simulink model "LWR"  (R2018b)
settings: Solver=FixedStepAuto  StartTime=0.0  StopTime=10  FixedStep=0.01  RelTol=1e-3
model workspace: external: MATLAB File F:\Research\AAA\LWR_DataFile.m (data not in the file)
values from neighbouring files (symbols this model uses):
  m = max([i j])    [Dynamic_model_eq.m]
  robot = robotics.RigidBodyTree("MaxNumBodies",8,"DataFormat","row")    [RigidBodyTree.m]
undefined symbols (not defined in the file or in its folder): smiData, X, Y, Z
libraries: sm_lib x86, fl_lib x42, nesl_utility x36, elec_lib x21, dspmtrx3 x7, robotmaniplib x2
(part 1 of 3)
settings Model: Creator=Cristian  LastModifiedBy=Cristian

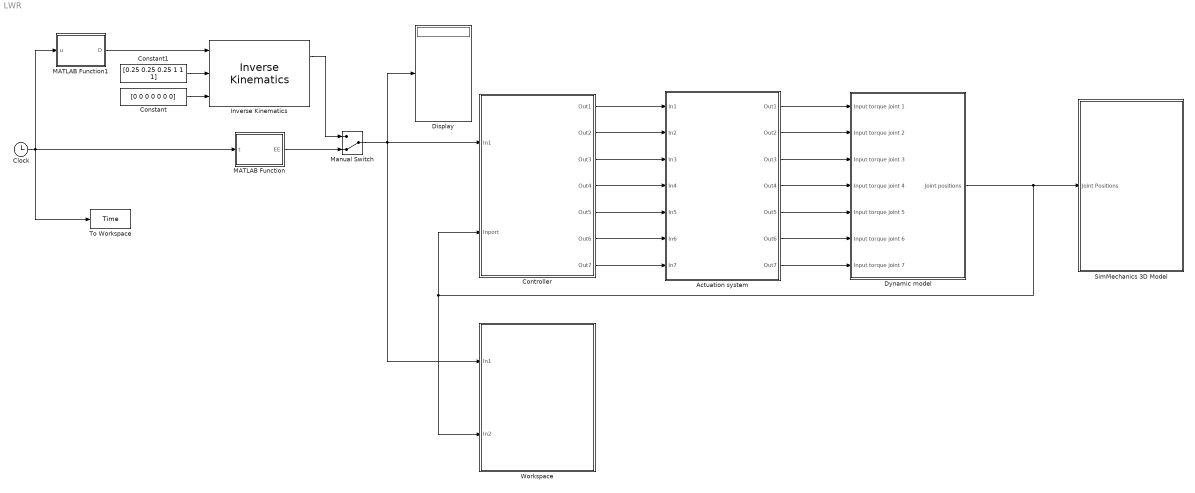
== system LWR ==
  Actuation system : Subsystem
  Clock : Clock
  Constant : Constant  Value=[0 0 0 0 0 0 0]
  Constant1 : Constant  Value=[0.25 0.25 0.25 1 1 1]
  Controller : Subsystem
  Display : Display
  "Dynamic model " : Subsystem
  Inverse Kinematics : robotmaniplib/Inverse Kinematics  RigidBodyTree=robot  EndEffector=body7  ShowInfo=on  SolverName=BFGS Gradient Projection  EnforceJointLimits=on  MaxIterations=1500  MaxTime=10  GradientTolerance=1e-7  SolutionTolerance=1e-6  StepTolerance=1e-14  ErrorChangeTolerance=1e-12  UseErrorDamping=on  DampingBias=0.0025
      settings: SourceProductName=Robotics System Toolbox
  MATLAB Function : MATLAB Function  TreatAsAtomicUnit=on
  MATLAB Function1 : MATLAB Function  TreatAsAtomicUnit=on
  Manual Switch : ManualSwitch  CurrentSetting=0
  SimMechanics 3D Model : Subsystem
      mask Display: image('photo1.jpg');
  To Workspace : ToWorkspace  VariableName=Time  SampleTime=-1
  Workspace : Subsystem
  wires:
  "Dynamic model "/1(Joint positions) -> Controller/2(Inport), Workspace/2(In2), SimMechanics 3D Model/1(Joint Positions)
  Controller/1(Out1) -> Actuation system/1(In1)
  Controller/2(Out2) -> Actuation system/2(In2)
  Controller/3(Out3) -> Actuation system/3(In3)
  Controller/4(Out4) -> Actuation system/4(In4)
  Controller/5(Out5) -> Actuation system/5(In5)
  Controller/6(Out6) -> Actuation system/6(In6)
  Controller/7(Out7) -> Actuation system/7(In7)
  Actuation system/1(Out1) -> "Dynamic model "/1(Input torque joint 1)
  Actuation system/2(Out2) -> "Dynamic model "/2(Input torque joint 2)
  Actuation system/3(Out3) -> "Dynamic model "/3(Input torque joint 3)
  Actuation system/4(Out4) -> "Dynamic model "/4(Input torque joint 4)
  Actuation system/5(Out5) -> "Dynamic model "/5(Input torque joint 5)
  Actuation system/6(Out6) -> "Dynamic model "/6(Input torque joint 6)
  Actuation system/7(Out7) -> "Dynamic model "/7(Input torque joint 7)
  Clock/1 -> To Workspace/1, MATLAB Function/1(t), MATLAB Function1/1(u)
  Manual Switch/1 -> Display/1, Workspace/1(In1), Controller/1(In1)
  MATLAB Function/1(EE) -> Manual Switch/2
  Constant/1 -> Inverse Kinematics/3
  Constant1/1 -> Inverse Kinematics/2
  MATLAB Function1/1(O) -> Inverse Kinematics/1
  Inverse Kinematics/1 -> Manual Switch/1

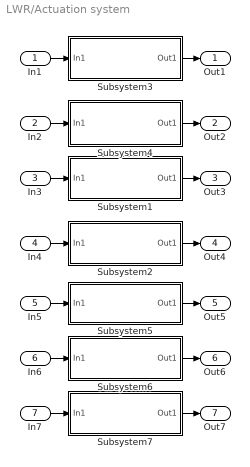
== system LWR/Actuation system ==
  In1 : Inport
  In2 : Inport  Port=2
  In3 : Inport  Port=3
  In4 : Inport  Port=4
  In5 : Inport  Port=5
  In6 : Inport  Port=6
  In7 : Inport  Port=7
  Subsystem1 : Subsystem
  Subsystem2 : Subsystem
  Subsystem3 : Subsystem
  Subsystem4 : Subsystem
  Subsystem5 : Subsystem
  Subsystem6 : Subsystem
  Subsystem7 : Subsystem
  Out1 : Outport
  Out2 : Outport  Port=2
  Out3 : Outport  Port=3
  Out4 : Outport  Port=4
  Out5 : Outport  Port=5
  Out6 : Outport  Port=6
  Out7 : Outport  Port=7
  wires:
  In2/1 -> Subsystem4/1(In1)
  In3/1 -> Subsystem1/1(In1)
  Subsystem7/1(Out1) -> Out7/1
  In1/1 -> Subsystem3/1(In1)
  In5/1 -> Subsystem5/1(In1)
  Subsystem1/1(Out1) -> Out3/1
  Subsystem5/1(Out1) -> Out5/1
  Subsystem4/1(Out1) -> Out2/1
  Subsystem3/1(Out1) -> Out1/1
  In6/1 -> Subsystem6/1(In1)
  Subsystem2/1(Out1) -> Out4/1
  Subsystem6/1(Out1) -> Out6/1
  In4/1 -> Subsystem2/1(In1)
  In7/1 -> Subsystem7/1(In1)

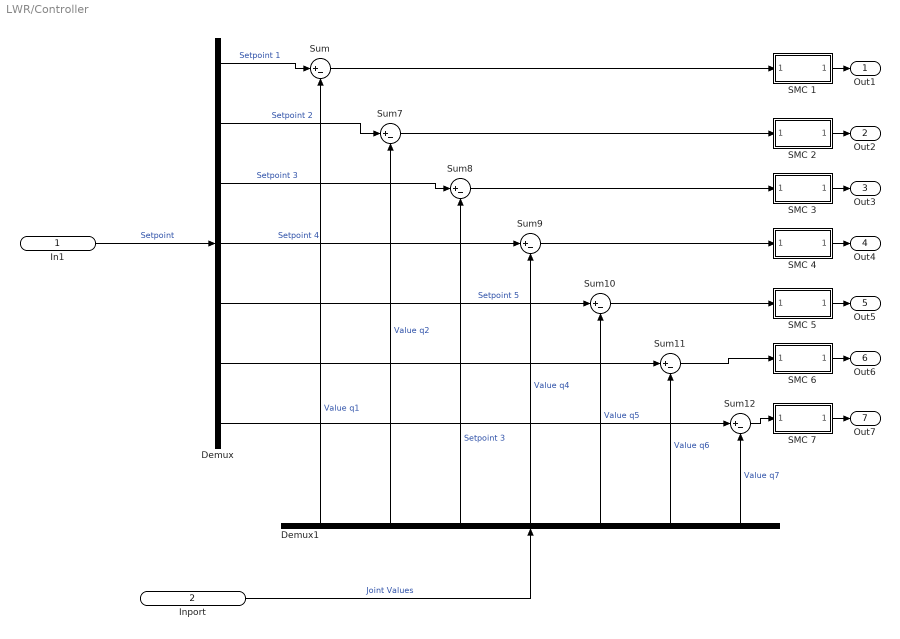
== system LWR/Controller ==
  In1 : Inport
  Inport : Inport  Port=2
  Demux : Demux  Outputs=7
  Demux1 : Demux  Outputs=7
  SMC 1 : Subsystem
  SMC 2 : Subsystem
  SMC 3 : Subsystem
  SMC 4 : Subsystem
  SMC 5 : Subsystem
  SMC 6 : Subsystem
  SMC 7 : Subsystem
  Sum{,7..12} (7 alike) : Sum  Inputs=|+-
  Out1 : Outport
  Out2 : Outport  Port=2
  Out3 : Outport  Port=3
  Out4 : Outport  Port=4
  Out5 : Outport  Port=5
  Out6 : Outport  Port=6
  Out7 : Outport  Port=7
  wires:
  Sum/1 -> SMC 1/1(error)
  Sum9/1 -> SMC 4/1(error)
  Sum8/1 -> SMC 3/1(error)
  Demux1/6 -> Sum11/2  "Value q6"
  Demux1/1 -> Sum/2  "Value q1"
  Demux/1 -> Sum/1  "Setpoint 1"
  Demux1/5 -> Sum10/2  "Value q5"
  Sum7/1 -> SMC 2/1(error)
  SMC 5/1(Out1) -> Out5/1
  Sum10/1 -> SMC 5/1(error)
  Sum11/1 -> SMC 6/1(error)
  Sum12/1 -> SMC 7/1(error)
  Demux/2 -> Sum7/1  "Setpoint 2"
  Demux/3 -> Sum8/1  "Setpoint 3"
  Demux1/4 -> Sum9/2  "Value q4"
  SMC 6/1(Out1) -> Out6/1
  SMC 4/1(Out1) -> Out4/1
  Demux/5 -> Sum10/1  "Setpoint 5"
  Demux1/2 -> Sum7/2  "Value q2"
  Demux1/3 -> Sum8/2  "Setpoint 3"
  Demux/4 -> Sum9/1  "Setpoint 4"
  SMC 2/1(Out1) -> Out2/1
  SMC 7/1(Out1) -> Out7/1
  Demux1/7 -> Sum12/2  "Value q7"
  SMC 3/1(Out1) -> Out3/1
  SMC 1/1(Out1) -> Out1/1
  Inport/1 -> Demux1/1  "Joint Values"
  In1/1 -> Demux/1  "Setpoint"
  Demux/6 -> Sum11/1
  Demux/7 -> Sum12/1

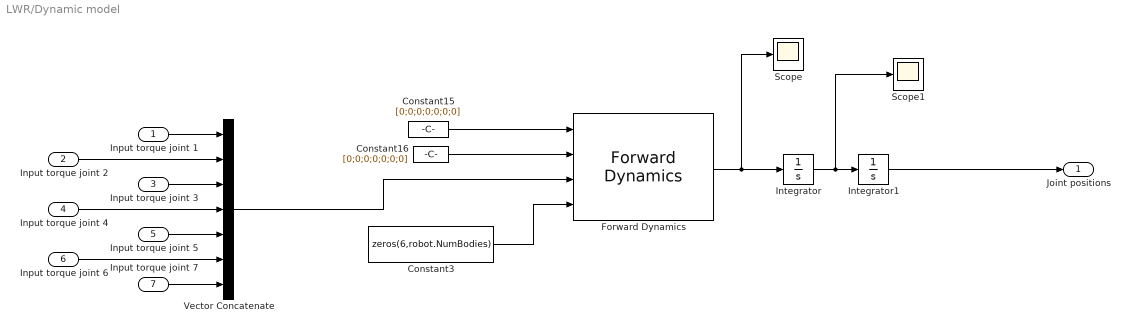
== system LWR/Dynamic model  ==
  Input torque joint 1 : Inport
  Input torque joint 2 : Inport  Port=2
  Input torque joint 3 : Inport  Port=3
  Input torque joint 4 : Inport  Port=4
  Input torque joint 5 : Inport  Port=5
  Input torque joint 6 : Inport  Port=6
  Input torque joint 7 : Inport  Port=7
  Constant15 : Constant  Value=[0;0;0;0;0;0;0]
  Constant16 : Constant  Value=[0;0;0;0;0;0;0]
  Constant3 : Constant  Value=zeros(6,robot.NumBodies)
  Forward Dynamics : robotmaniplib/Forward Dynamics  RigidBodyTree=robot
      settings: SourceProductName=Robotics System Toolbox
  Integrator : Integrator
  Integrator1 : Integrator
  Scope : Scope
  Scope1 : Scope
  Vector Concatenate : Concatenate  NumInputs=7
  Joint positions : Outport
  wires:
  Constant16/1 -> Forward Dynamics/2
  Forward Dynamics/1 -> Scope/1, Integrator/1
  Constant15/1 -> Forward Dynamics/1
  Integrator/1 -> Scope1/1, Integrator1/1
  Integrator1/1 -> Joint positions/1
  Vector Concatenate/1 -> Forward Dynamics/3
  Constant3/1 -> Forward Dynamics/4
  Input torque joint 1/1 -> Vector Concatenate/1
  Input torque joint 2/1 -> Vector Concatenate/2
  Input torque joint 3/1 -> Vector Concatenate/3
  Input torque joint 4/1 -> Vector Concatenate/4
  Input torque joint 5/1 -> Vector Concatenate/5
  Input torque joint 6/1 -> Vector Concatenate/6
  Input torque joint 7/1 -> Vector Concatenate/7

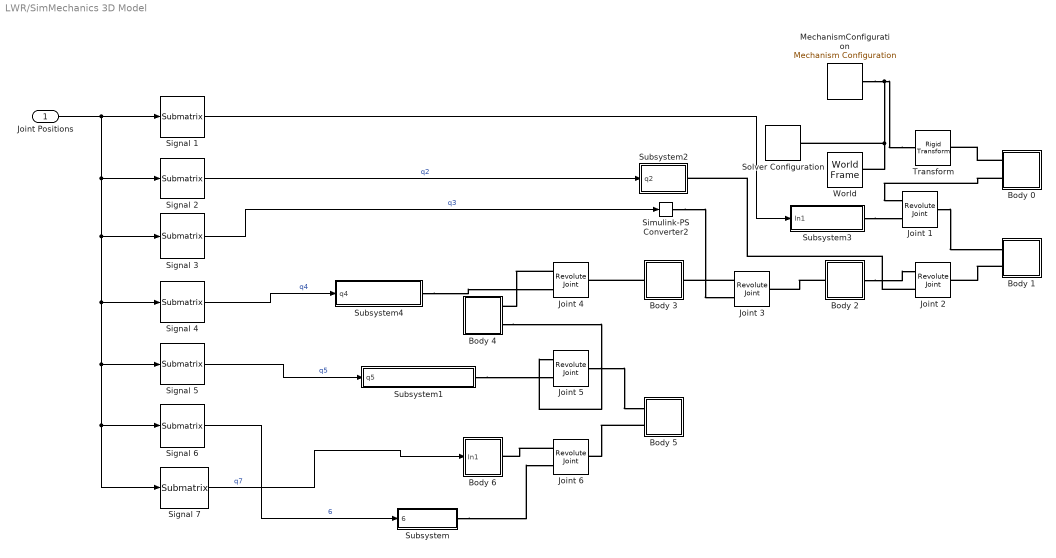
== system LWR/SimMechanics 3D Model ==
  Joint Positions : Inport
  Body 0 : Subsystem
  Body 1 : Subsystem
  Body 2 : Subsystem
  Body 3 : Subsystem
  Body 4 : Subsystem
  Body 5 : Subsystem
  Body 6 : Subsystem
  Joint 1 : sm_lib/Joints/Revolute Joint  SenseConstraintForce=off  SenseConstraintForceX=off  SenseConstraintForceY=off  SenseConstraintForceZ=off  SenseConstraintTorque=off  SenseConstraintTorqueX=off  SenseConstraintTorqueY=off  SenseConstraintTorqueZ=off  SenseTotalForce=off  SenseTotalForceX=off  SenseTotalForceY=off  SenseTotalForceZ=off  SenseTotalTorque=off  SenseTotalTorqueX=off  SenseTotalTorqueY=off  SenseTotalTorqueZ=off  CompositeWrenchDir=FollowerOnBase  CompositeWrenchFrame=BaseFrame  EquilibriumPosition=0  EquilibriumPositionUnits=rad  SpringStiffness=0  SpringStiffnessUnits=N*m/rad  DampingCoefficient=0  DampingCoefficientUnits=N*m/(rad/s)  TorqueActuationMode=ComputedTorque  MotionActuationMode=InputMotion  SensePosition=off  SenseVelocity=off  SenseAcceleration=off  SenseTorqueForce=off  PositionTargetSpecify=on  PositionTargetPriority=High  PositionTargetValue=2.094395  PositionTargetValueUnits=rad  VelocityTargetSpecify=on  VelocityTargetPriority=High  VelocityTargetValue=0  VelocityTargetValueUnits=deg/s
  Joint 2 : sm_lib/Joints/Revolute Joint  SenseConstraintForce=off  SenseConstraintForceX=off  SenseConstraintForceY=off  SenseConstraintForceZ=off  SenseConstraintTorque=off  SenseConstraintTorqueX=off  SenseConstraintTorqueY=off  SenseConstraintTorqueZ=off  SenseTotalForce=off  SenseTotalForceX=off  SenseTotalForceY=off  SenseTotalForceZ=off  SenseTotalTorque=off  SenseTotalTorqueX=off  SenseTotalTorqueY=off  SenseTotalTorqueZ=off  CompositeWrenchDir=FollowerOnBase  CompositeWrenchFrame=BaseFrame  EquilibriumPosition=0  EquilibriumPositionUnits=rad  SpringStiffness=0  SpringStiffnessUnits=N*m/rad  DampingCoefficient=0  DampingCoefficientUnits=N*m/(rad/s)  TorqueActuationMode=ComputedTorque  MotionActuationMode=InputMotion  SensePosition=off  SenseVelocity=off  SenseAcceleration=off  SenseTorqueForce=off  PositionTargetSpecify=on  PositionTargetPriority=High  PositionTargetValue=5.9341  PositionTargetValueUnits=rad  VelocityTargetSpecify=on  VelocityTargetPriority=High  VelocityTargetValue=0  VelocityTargetValueUnits=deg/s
  Joint 3 : sm_lib/Joints/Revolute Joint  SenseConstraintForce=off  SenseConstraintForceX=off  SenseConstraintForceY=off  SenseConstraintForceZ=off  SenseConstraintTorque=off  SenseConstraintTorqueX=off  SenseConstraintTorqueY=off  SenseConstraintTorqueZ=off  SenseTotalForce=off  SenseTotalForceX=off  SenseTotalForceY=off  SenseTotalForceZ=off  SenseTotalTorque=off  SenseTotalTorqueX=off  SenseTotalTorqueY=off  SenseTotalTorqueZ=off  CompositeWrenchDir=FollowerOnBase  CompositeWrenchFrame=BaseFrame  EquilibriumPosition=0  EquilibriumPositionUnits=rad  SpringStiffness=0  SpringStiffnessUnits=N*m/rad  DampingCoefficient=0  DampingCoefficientUnits=N*m/(rad/s)  TorqueActuationMode=ComputedTorque  MotionActuationMode=InputMotion  SensePosition=off  SenseVelocity=off  SenseAcceleration=off  SenseTorqueForce=off  PositionTargetSpecify=on  PositionTargetPriority=High  PositionTargetValue=0  PositionTargetValueUnits=deg  VelocityTargetSpecify=off  VelocityTargetPriority=High  VelocityTargetValue=0  VelocityTargetValueUnits=deg/s
  Joint 4 : sm_lib/Joints/Revolute Joint  SenseConstraintForce=off  SenseConstraintForceX=off  SenseConstraintForceY=off  SenseConstraintForceZ=off  SenseConstraintTorque=off  SenseConstraintTorqueX=off  SenseConstraintTorqueY=off  SenseConstraintTorqueZ=off  SenseTotalForce=off  SenseTotalForceX=off  SenseTotalForceY=off  SenseTotalForceZ=off  SenseTotalTorque=off  SenseTotalTorqueX=off  SenseTotalTorqueY=off  SenseTotalTorqueZ=off  CompositeWrenchDir=FollowerOnBase  CompositeWrenchFrame=BaseFrame  EquilibriumPosition=0  EquilibriumPositionUnits=rad  SpringStiffness=0  SpringStiffnessUnits=N*m/rad  DampingCoefficient=0  DampingCoefficientUnits=N*m/(rad/s)  TorqueActuationMode=ComputedTorque  MotionActuationMode=InputMotion  SensePosition=off  SenseVelocity=off  SenseAcceleration=off  SenseTorqueForce=off  PositionTargetSpecify=on  PositionTargetPriority=High  PositionTargetValue=4.8869  PositionTargetValueUnits=rad  VelocityTargetSpecify=off  VelocityTargetPriority=High  VelocityTargetValue=0  VelocityTargetValueUnits=deg/s
  Joint 5 : sm_lib/Joints/Revolute Joint  SenseConstraintForce=off  SenseConstraintForceX=off  SenseConstraintForceY=off  SenseConstraintForceZ=off  SenseConstraintTorque=off  SenseConstraintTorqueX=off  SenseConstraintTorqueY=off  SenseConstraintTorqueZ=off  SenseTotalForce=off  SenseTotalForceX=off  SenseTotalForceY=off  SenseTotalForceZ=off  SenseTotalTorque=off  SenseTotalTorqueX=off  SenseTotalTorqueY=off  SenseTotalTorqueZ=off  CompositeWrenchDir=FollowerOnBase  CompositeWrenchFrame=BaseFrame  EquilibriumPosition=0  EquilibriumPositionUnits=rad  SpringStiffness=0  SpringStiffnessUnits=N*m/rad  DampingCoefficient=0  DampingCoefficientUnits=N*m/(rad/s)  TorqueActuationMode=ComputedTorque  MotionActuationMode=InputMotion  SensePosition=off  SenseVelocity=off  SenseAcceleration=off  SenseTorqueForce=off  PositionTargetSpecify=on  PositionTargetPriority=High  PositionTargetValue=0.349  PositionTargetValueUnits=rad  VelocityTargetSpecify=off  VelocityTargetPriority=High  VelocityTargetValue=0  VelocityTargetValueUnits=deg/s
  Joint 6 : sm_lib/Joints/Revolute Joint  SenseConstraintForce=off  SenseConstraintForceX=off  SenseConstraintForceY=off  SenseConstraintForceZ=off  SenseConstraintTorque=off  SenseConstraintTorqueX=off  SenseConstraintTorqueY=off  SenseConstraintTorqueZ=off  SenseTotalForce=off  SenseTotalForceX=off  SenseTotalForceY=off  SenseTotalForceZ=off  SenseTotalTorque=off  SenseTotalTorqueX=off  SenseTotalTorqueY=off  SenseTotalTorqueZ=off  CompositeWrenchDir=FollowerOnBase  CompositeWrenchFrame=BaseFrame  EquilibriumPosition=0  EquilibriumPositionUnits=rad  SpringStiffness=0  SpringStiffnessUnits=N*m/rad  DampingCoefficient=0  DampingCoefficientUnits=N*m/(rad/s)  TorqueActuationMode=ComputedTorque  MotionActuationMode=InputMotion  SensePosition=off  SenseVelocity=off  SenseAcceleration=off  SenseTorqueForce=off  PositionTargetSpecify=on  PositionTargetPriority=Low  PositionTargetValue=0.2617  PositionTargetValueUnits=rad  VelocityTargetSpecify=off  VelocityTargetPriority=High  VelocityTargetValue=0  VelocityTargetValueUnits=deg/s
  MechanismConfiguration : sm_lib/Utilities/Mechanism Configuration  UniformGravity=Constant  GravityVector=[0 -9.80665 0]  GravityUnits=m/s^2  LinearizationDelta=0.001
  Signal 1 : dspmtrx3/Submatrix  RowSpan=One row  RowStartMode=First  RowStartIndex=1  RowEndMode=Last  RowEndIndex=1  ColSpan=One column  ColStartMode=First  ColStartIndex=1  ColEndMode=Last  ColEndIndex=1
  Signal 2 : dspmtrx3/Submatrix  RowSpan=One row  RowStartMode=Index  RowStartIndex=2  RowEndMode=Last  RowEndIndex=1  ColSpan=One column  ColStartMode=First  ColStartIndex=1  ColEndMode=Last  ColEndIndex=1
  Signal 3 : dspmtrx3/Submatrix  RowSpan=One row  RowStartMode=Index  RowStartIndex=3  RowEndMode=Last  RowEndIndex=1  ColSpan=One column  ColStartMode=First  ColStartIndex=1  ColEndMode=Last  ColEndIndex=1
  Signal 4 : dspmtrx3/Submatrix  RowSpan=One row  RowStartMode=Index  RowStartIndex=4  RowEndMode=Last  RowEndIndex=1  ColSpan=One column  ColStartMode=First  ColStartIndex=1  ColEndMode=Last  ColEndIndex=1
  Signal 5 : dspmtrx3/Submatrix  RowSpan=One row  RowStartMode=Index  RowStartIndex=5  RowEndMode=Last  RowEndIndex=1  ColSpan=One column  ColStartMode=First  ColStartIndex=1  ColEndMode=Last  ColEndIndex=1
  Signal 6 : dspmtrx3/Submatrix  RowSpan=One row  RowStartMode=Index  RowStartIndex=6  RowEndMode=Last  RowEndIndex=1  ColSpan=One column  ColStartMode=First  ColStartIndex=1  ColEndMode=Last  ColEndIndex=1
  Signal 7 : dspmtrx3/Submatrix  RowSpan=One row  RowStartMode=Index  RowStartIndex=7  RowEndMode=Last  RowEndIndex=1  ColSpan=One column  ColStartMode=First  ColStartIndex=1  ColEndMode=Last  ColEndIndex=1
  Simulink-PS Converter2 : nesl_utility/Simulink-PS Converter  PhysicalDomain=network_engine_domain  SubClassName=ps_input  LeftPortType=input  RightPortType=output  PseudoPeriodic=off  Frequencies=[]  NoiseDistribution=none  NoiseParameters=[]  Unit=rad  AffineConversion=off  FilteringAndDerivatives=filter  SimscapeFilterOrder=2  InputFilterTimeConstant=0.001  UdotUserProvided=0
  Solver Configuration : nesl_utility/Solver Configuration  PhysicalDomain=network_engine_domain  SubClassName=solver  LeftPortType=input  RightPortType=generic  Tones=[]  Harmonics=[]  SimulateNoise=off  Profile=off  UseLocalSampling=off  EnableSwitchedLinearOptims=on  FrequencyDomain=off  UseCCode=off  RelTol=0.001  AbsTol=1e-06  MinStep=1e-09  ToWorkspace=off  RevertToSquareIcSolve=off  NumHomotopyIterations=100  PhasorMode=off  PhasorModeNumHarmonics=1  DoDC=off  ResidualTolerance=1e-09  UseLocalSolver=off  LocalSolverChoice=NE_BACKWARD_EULER_ADVANCER  LocalSolverSampleTime=0.001  DoFixedCost=off  MaxNonlinIter=3  MaxModeIter=2  LinearAlgebra=auto  EquationFormulation=NE_TIME_EF  DelaysMemoryBudget=1024  AutomaticFiltering=on  FilteringTimeConstant=0.001  PartitionStorageMethod=AS_NEEDED  PartitionMemoryBudget=1024
  Subsystem : Subsystem
  Subsystem1 : Subsystem
  Subsystem2 : Subsystem
  Subsystem3 : Subsystem
  Subsystem4 : Subsystem
  Transform : sm_lib/Frames and Transforms/Rigid Transform  TranslationMethod=Cartesian  TranslationStandardOffset=0  TranslationLengthUnit=mm  TranslationStandardAxis=+Z  TranslationCartesianOffset=smiData.RigidTransform(32).translation  TranslationROffset=0  TranslationROffsetUnits=m  TranslationZOffset=0  TranslationZOffsetUnits=m  TranslationThetaOffset=0  TranslationThetaOffsetUnits=deg  RotationMethod=None  RotationAngleUnits=deg  RotationStandardAxis=+Z  RotationAngle=90  RotationArbitraryAxis=smiData.RigidTransform(32).axis  FollAlignAxisA=+X  BaseAlignAxisA=+Y  FollAlignAxisB=+Y  BaseAlignAxisB=+Z  RotationSequenceAxes=FollowerAxes  RotationSequence=XYX  RotationSequenceAngles=[0 0 0]  RotationSequenceAnglesUnits=deg  RotationMatrix=[1 0 0; 0 1 0; 0 0 1]
  World : sm_lib/Frames and Transforms/World Frame
  wires:
  Signal 3/1 -> Simulink-PS Converter2/1  "q3"
  Signal 7/1 -> Body 6/1(In1)  "q7"
  Joint Positions/1 -> Signal 2/1, Signal 3/1, Signal 5/1, Signal 6/1, Signal 7/1, Signal 4/1, Signal 1/1
  Signal 6/1 -> Subsystem/1(6)  "6"
  Signal 5/1 -> Subsystem1/1(q5)  "q5"
  Signal 2/1 -> Subsystem2/1(q2)  "q2"
  Signal 1/1 -> Subsystem3/1(In1)
  Signal 4/1 -> Subsystem4/1(q4)  "q4"
  connections:
  Transform/LConn1 -- MechanismConfiguration/RConn1 -- Solver Configuration/RConn1 -- World/RConn1
  Body 1/LConn2 -- Joint 2/RConn1
  Body 0/LConn1 -- Transform/RConn1
  Body 2/RConn1 -- Joint 2/LConn1
  Simulink-PS Converter2/RConn1 -- Joint 3/LConn2
  Body 0/LConn2 -- Joint 1/LConn1
  Joint 1/RConn1 -- Body 1/LConn1
  Body 2/LConn1 -- Joint 3/RConn1
  Joint 3/LConn1 -- Body 3/RConn1
  Body 3/LConn1 -- Joint 4/RConn1
  Joint 4/LConn1 -- Body 4/RConn1
  Body 4/RConn2 -- Joint 5/LConn1
  Joint 5/RConn1 -- Body 5/LConn1
  Body 5/LConn2 -- Joint 6/RConn1
  Joint 6/LConn1 -- Body 6/RConn1
  Subsystem/RConn1 -- Joint 6/LConn2
  Subsystem1/RConn1 -- Joint 5/LConn2
  Joint 2/LConn2 -- Subsystem2/RConn1
  Subsystem3/RConn1 -- Joint 1/LConn2
  Subsystem4/RConn1 -- Joint 4/LConn2

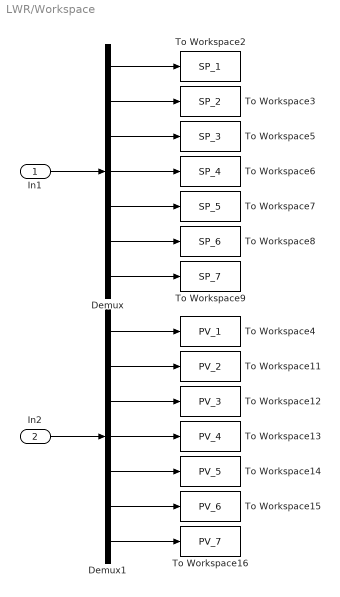
== system LWR/Workspace ==
  In1 : Inport
  In2 : Inport  Port=2
  Demux : Demux  Outputs=7
  Demux1 : Demux  Outputs=7
  To Workspace11 : ToWorkspace  VariableName=PV_2  SampleTime=-1
  To Workspace12 : ToWorkspace  VariableName=PV_3  SampleTime=-1
  To Workspace13 : ToWorkspace  VariableName=PV_4  SampleTime=-1
  To Workspace14 : ToWorkspace  VariableName=PV_5  SampleTime=-1
  To Workspace15 : ToWorkspace  VariableName=PV_6  SampleTime=-1
  To Workspace16 : ToWorkspace  VariableName=PV_7  SampleTime=-1
  To Workspace2 : ToWorkspace  VariableName=SP_1  SampleTime=-1
  To Workspace3 : ToWorkspace  VariableName=SP_2  SampleTime=-1
  To Workspace4 : ToWorkspace  VariableName=PV_1  SampleTime=-1
  To Workspace5 : ToWorkspace  VariableName=SP_3  SampleTime=-1
  To Workspace6 : ToWorkspace  VariableName=SP_4  SampleTime=-1
  To Workspace7 : ToWorkspace  VariableName=SP_5  SampleTime=-1
  To Workspace8 : ToWorkspace  VariableName=SP_6  SampleTime=-1
  To Workspace9 : ToWorkspace  VariableName=SP_7  SampleTime=-1
  wires:
  In1/1 -> Demux/1
  In2/1 -> Demux1/1
  Demux/1 -> To Workspace2/1
  Demux/2 -> To Workspace3/1
  Demux/3 -> To Workspace5/1
  Demux/4 -> To Workspace6/1
  Demux/7 -> To Workspace9/1
  Demux/6 -> To Workspace8/1
  Demux/5 -> To Workspace7/1
  Demux1/1 -> To Workspace4/1
  Demux1/7 -> To Workspace16/1
  Demux1/6 -> To Workspace15/1
  Demux1/5 -> To Workspace14/1
  Demux1/4 -> To Workspace13/1
  Demux1/3 -> To Workspace12/1
  Demux1/2 -> To Workspace11/1

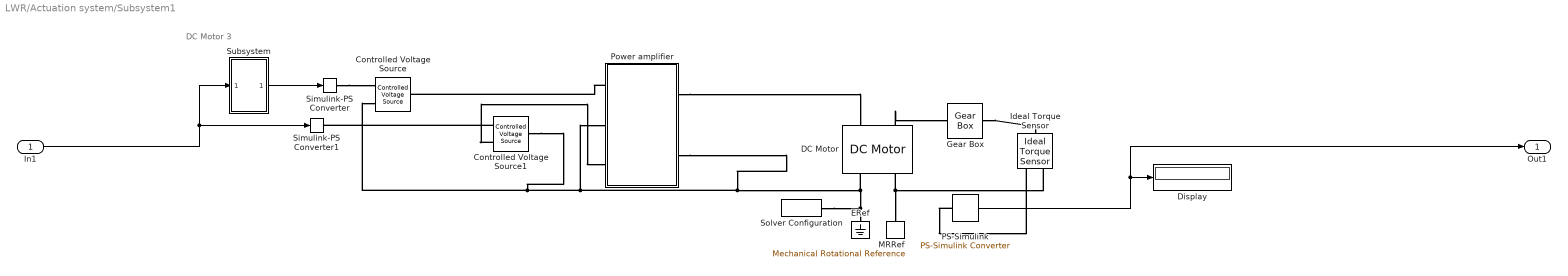
== system LWR/Actuation system/Subsystem1 ==
  note: DC Motor 3
  In1 : Inport
  Controlled Voltage Source : fl_lib/Electrical/Electrical Sources/Controlled Voltage Source
  Controlled Voltage Source1 : fl_lib/Electrical/Electrical Sources/Controlled Voltage Source
  DC Motor : elec_lib/Actuators & Drivers/Rotational Actuators/DC Motor  parameterization=1  Ra=3.38 Ohm  La=0.01 H  emf_or_torque=2  Kv=0.029 V/(rad/s)  Ki=0.638 N*m/A  T_stall=0.1 N*m  w_max=4000 rpm  w_rated=2500 rpm  P_rated=10 W  V_rated=12 V  J=0.2 kg*m^2  lam_param=1  lam=0.5e-5 N*m/(rad/s)  i_noload=0 A  V_i_noload=1.5 V  speed0=0 rpm  alpha=0.00393 1/K  Tmeas=25 degC  thermal_mass=100 J/K  initial_temperature=25 degC
  Display : Display
  ERef : fl_lib/Electrical/Electrical Elements/Electrical Reference
      settings: SourceProductName=Foundation Library
  Gear Box : fl_lib/Mechanical/Mechanisms/Gear Box  ratio=2.5  t_in_specify=off  t_in_priority=None  t_in=0 N*m  t_in_nominal_specify=off  t_in_nominal_unit=N*m  t_in_nominal_value=1  t_out_specify=off  t_out_priority=None  t_out=0 N*m  t_out_nominal_specify=off  t_out_nominal_unit=N*m  t_out_nominal_value=1
  Ideal Torque Sensor : fl_lib/Mechanical/Mechanical Sensors/Ideal Torque Sensor
  MRRef : fl_lib/Mechanical/Rotational Elements/Mechanical Rotational Reference
      settings: SourceProductName=Foundation Library
  PS-Simulink : nesl_utility/PS-Simulink Converter  PhysicalDomain=network_engine_domain  SubClassName=ps_output  LeftPortType=input  RightPortType=output  PseudoPeriodic=off  Frequencies=[]  Unit=N*m  AffineConversion=off
  Power amplifier : Subsystem
  Simulink-PS Converter : nesl_utility/Simulink-PS Converter  PhysicalDomain=network_engine_domain  SubClassName=ps_input  LeftPortType=input  RightPortType=output  PseudoPeriodic=off  Frequencies=[]  NoiseDistribution=none  NoiseParameters=[]  Unit=V  AffineConversion=off  FilteringAndDerivatives=provide  SimscapeFilterOrder=1  InputFilterTimeConstant=0.001  UdotUserProvided=0
  Simulink-PS Converter1 : nesl_utility/Simulink-PS Converter  PhysicalDomain=network_engine_domain  SubClassName=ps_input  LeftPortType=input  RightPortType=output  PseudoPeriodic=off  Frequencies=[]  NoiseDistribution=none  NoiseParameters=[]  Unit=V  AffineConversion=off  FilteringAndDerivatives=provide  SimscapeFilterOrder=1  InputFilterTimeConstant=0.001  UdotUserProvided=0
  Solver Configuration : nesl_utility/Solver Configuration  PhysicalDomain=network_engine_domain  SubClassName=solver  LeftPortType=input  RightPortType=generic  Tones=[]  Harmonics=[]  SimulateNoise=off  Profile=off  UseLocalSampling=off  EnableSwitchedLinearOptims=on  FrequencyDomain=off  UseCCode=off  RelTol=0.001  AbsTol=1e-06  MinStep=1e-09  ToWorkspace=off  RevertToSquareIcSolve=off  NumHomotopyIterations=100  PhasorMode=off  PhasorModeNumHarmonics=1  DoDC=off  ResidualTolerance=1e-9  UseLocalSolver=off  LocalSolverChoice=NE_BACKWARD_EULER_ADVANCER  LocalSolverSampleTime=.001  DoFixedCost=off  MaxNonlinIter=3  MaxModeIter=2  LinearAlgebra=auto  EquationFormulation=NE_TIME_EF  DelaysMemoryBudget=1024  AutomaticFiltering=on  FilteringTimeConstant=0.001  PartitionStorageMethod=AS_NEEDED  PartitionMemoryBudget=1024
  Subsystem : Subsystem
  Out1 : Outport
  wires:
  PS-Simulink/1 -> Out1/1, Display/1
  Subsystem/1(Out1) -> Simulink-PS Converter/1
  In1/1 -> Subsystem/1(In1), Simulink-PS Converter1/1
  connections:
  DC Motor/LConn2 -- Gear Box/LConn1
  Power amplifier/LConn1 -- Controlled Voltage Source/LConn1
  Gear Box/RConn1 -- Ideal Torque Sensor/LConn1
  Controlled Voltage Source1/RConn1 -- Simulink-PS Converter1/RConn1
  DC Motor/RConn2 -- Ideal Torque Sensor/RConn1 -- MRRef/LConn1
  Controlled Voltage Source1/RConn2 -- Power amplifier/LConn3
  DC Motor/RConn1 -- Power amplifier/RConn2 -- Controlled Voltage Source1/LConn1 -- Controlled Voltage Source/RConn2 -- Power amplifier/LConn2 -- Solver Configuration/RConn1 -- ERef/LConn1
  Simulink-PS Converter/RConn1 -- Controlled Voltage Source/RConn1
  PS-Simulink/LConn1 -- Ideal Torque Sensor/RConn2
  Power amplifier/RConn1 -- DC Motor/LConn1

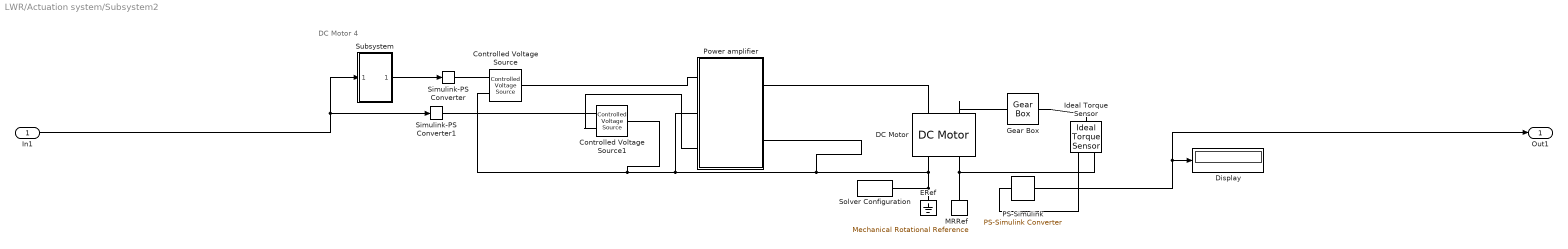
== system LWR/Actuation system/Subsystem2 ==
  note: DC Motor 4
  In1 : Inport
  Controlled Voltage Source : fl_lib/Electrical/Electrical Sources/Controlled Voltage Source
  Controlled Voltage Source1 : fl_lib/Electrical/Electrical Sources/Controlled Voltage Source
  DC Motor : elec_lib/Actuators & Drivers/Rotational Actuators/DC Motor  parameterization=1  Ra=3.38 Ohm  La=0.01 H  emf_or_torque=2  Kv=0.029 V/(rad/s)  Ki=0.638 N*m/A  T_stall=0.1 N*m  w_max=4000 rpm  w_rated=2500 rpm  P_rated=10 W  V_rated=12 V  J=0.2 kg*m^2  lam_param=1  lam=0.5e-5 N*m/(rad/s)  i_noload=0 A  V_i_noload=1.5 V  speed0=0 rpm  alpha=0.00393 1/K  Tmeas=25 degC  thermal_mass=100 J/K  initial_temperature=25 degC
  Display : Display
  ERef : fl_lib/Electrical/Electrical Elements/Electrical Reference
      settings: SourceProductName=Foundation Library
  Gear Box : fl_lib/Mechanical/Mechanisms/Gear Box  ratio=2.5  t_in_specify=off  t_in_priority=None  t_in=0 N*m  t_in_nominal_specify=off  t_in_nominal_unit=N*m  t_in_nominal_value=1  t_out_specify=off  t_out_priority=None  t_out=0 N*m  t_out_nominal_specify=off  t_out_nominal_unit=N*m  t_out_nominal_value=1
  Ideal Torque Sensor : fl_lib/Mechanical/Mechanical Sensors/Ideal Torque Sensor
  MRRef : fl_lib/Mechanical/Rotational Elements/Mechanical Rotational Reference
      settings: SourceProductName=Foundation Library
  PS-Simulink : nesl_utility/PS-Simulink Converter  PhysicalDomain=network_engine_domain  SubClassName=ps_output  LeftPortType=input  RightPortType=output  PseudoPeriodic=off  Frequencies=[]  Unit=N*m  AffineConversion=off
  Power amplifier : Subsystem
  Simulink-PS Converter : nesl_utility/Simulink-PS Converter  PhysicalDomain=network_engine_domain  SubClassName=ps_input  LeftPortType=input  RightPortType=output  PseudoPeriodic=off  Frequencies=[]  NoiseDistribution=none  NoiseParameters=[]  Unit=V  AffineConversion=off  FilteringAndDerivatives=provide  SimscapeFilterOrder=1  InputFilterTimeConstant=0.001  UdotUserProvided=0
  Simulink-PS Converter1 : nesl_utility/Simulink-PS Converter  PhysicalDomain=network_engine_domain  SubClassName=ps_input  LeftPortType=input  RightPortType=output  PseudoPeriodic=off  Frequencies=[]  NoiseDistribution=none  NoiseParameters=[]  Unit=V  AffineConversion=off  FilteringAndDerivatives=provide  SimscapeFilterOrder=1  InputFilterTimeConstant=0.001  UdotUserProvided=0
  Solver Configuration : nesl_utility/Solver Configuration  PhysicalDomain=network_engine_domain  SubClassName=solver  LeftPortType=input  RightPortType=generic  Tones=[]  Harmonics=[]  SimulateNoise=off  Profile=off  UseLocalSampling=off  EnableSwitchedLinearOptims=on  FrequencyDomain=off  UseCCode=off  RelTol=0.001  AbsTol=1e-06  MinStep=1e-09  ToWorkspace=off  RevertToSquareIcSolve=off  NumHomotopyIterations=100  PhasorMode=off  PhasorModeNumHarmonics=1  DoDC=off  ResidualTolerance=1e-9  UseLocalSolver=off  LocalSolverChoice=NE_BACKWARD_EULER_ADVANCER  LocalSolverSampleTime=.001  DoFixedCost=off  MaxNonlinIter=3  MaxModeIter=2  LinearAlgebra=auto  EquationFormulation=NE_TIME_EF  DelaysMemoryBudget=1024  AutomaticFiltering=on  FilteringTimeConstant=0.001  PartitionStorageMethod=AS_NEEDED  PartitionMemoryBudget=1024
  Subsystem : Subsystem
  Out1 : Outport
  wires:
  PS-Simulink/1 -> Out1/1, Display/1
  Subsystem/1(Out1) -> Simulink-PS Converter/1
  In1/1 -> Subsystem/1(In1), Simulink-PS Converter1/1
  connections:
  DC Motor/LConn2 -- Gear Box/LConn1
  Power amplifier/LConn1 -- Controlled Voltage Source/LConn1
  Gear Box/RConn1 -- Ideal Torque Sensor/LConn1
  Controlled Voltage Source1/RConn1 -- Simulink-PS Converter1/RConn1
  DC Motor/RConn2 -- Ideal Torque Sensor/RConn1 -- MRRef/LConn1
  Controlled Voltage Source1/RConn2 -- Power amplifier/LConn3
  DC Motor/RConn1 -- Power amplifier/RConn2 -- Controlled Voltage Source1/LConn1 -- Controlled Voltage Source/RConn2 -- Power amplifier/LConn2 -- Solver Configuration/RConn1 -- ERef/LConn1
  Power amplifier/RConn1 -- DC Motor/LConn1
  Simulink-PS Converter/RConn1 -- Controlled Voltage Source/RConn1
  PS-Simulink/LConn1 -- Ideal Torque Sensor/RConn2

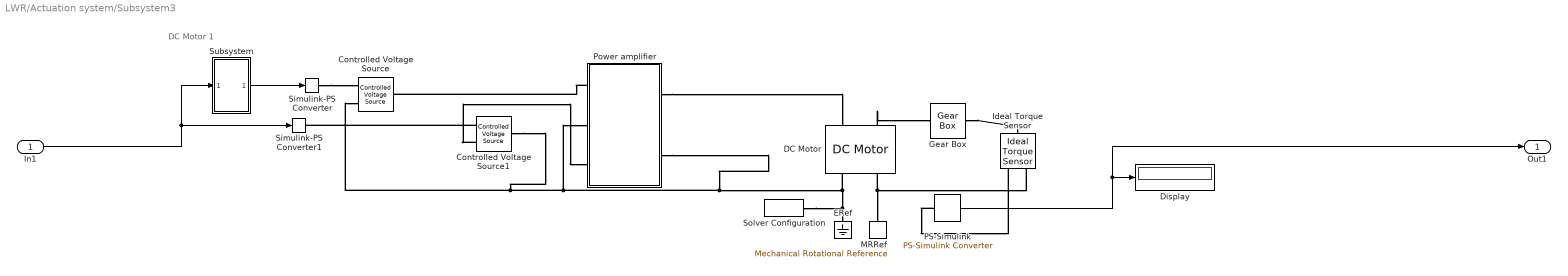
== system LWR/Actuation system/Subsystem3 ==
  note: DC Motor 1
  In1 : Inport
  Controlled Voltage Source : fl_lib/Electrical/Electrical Sources/Controlled Voltage Source
  Controlled Voltage Source1 : fl_lib/Electrical/Electrical Sources/Controlled Voltage Source
  DC Motor : elec_lib/Actuators & Drivers/Rotational Actuators/DC Motor  parameterization=1  Ra=3.38 Ohm  La=0.01 H  emf_or_torque=2  Kv=0.029 V/(rad/s)  Ki=0.638 N*m/A  T_stall=0.1 N*m  w_max=4000 rpm  w_rated=2500 rpm  P_rated=10 W  V_rated=12 V  J=0.2 kg*m^2  lam_param=1  lam=0.5e-5 N*m/(rad/s)  i_noload=0 A  V_i_noload=1.5 V  speed0=0 rpm  alpha=0.00393 1/K  Tmeas=25 degC  thermal_mass=100 J/K  initial_temperature=25 degC
  Display : Display
  ERef : fl_lib/Electrical/Electrical Elements/Electrical Reference
      settings: SourceProductName=Foundation Library
  Gear Box : fl_lib/Mechanical/Mechanisms/Gear Box  ratio=4  t_in_specify=off  t_in_priority=None  t_in=0 N*m  t_in_nominal_specify=off  t_in_nominal_unit=N*m  t_in_nominal_value=1  t_out_specify=off  t_out_priority=None  t_out=0 N*m  t_out_nominal_specify=off  t_out_nominal_unit=N*m  t_out_nominal_value=1
  Ideal Torque Sensor : fl_lib/Mechanical/Mechanical Sensors/Ideal Torque Sensor
  MRRef : fl_lib/Mechanical/Rotational Elements/Mechanical Rotational Reference
      settings: SourceProductName=Foundation Library
  PS-Simulink : nesl_utility/PS-Simulink Converter  PhysicalDomain=network_engine_domain  SubClassName=ps_output  LeftPortType=input  RightPortType=output  PseudoPeriodic=off  Frequencies=[]  Unit=N*m  AffineConversion=off
  Power amplifier : Subsystem
  Simulink-PS Converter : nesl_utility/Simulink-PS Converter  PhysicalDomain=network_engine_domain  SubClassName=ps_input  LeftPortType=input  RightPortType=output  PseudoPeriodic=off  Frequencies=[]  NoiseDistribution=none  NoiseParameters=[]  Unit=V  AffineConversion=off  FilteringAndDerivatives=provide  SimscapeFilterOrder=1  InputFilterTimeConstant=0.001  UdotUserProvided=0
  Simulink-PS Converter1 : nesl_utility/Simulink-PS Converter  PhysicalDomain=network_engine_domain  SubClassName=ps_input  LeftPortType=input  RightPortType=output  PseudoPeriodic=off  Frequencies=[]  NoiseDistribution=none  NoiseParameters=[]  Unit=V  AffineConversion=off  FilteringAndDerivatives=provide  SimscapeFilterOrder=1  InputFilterTimeConstant=0.001  UdotUserProvided=0
  Solver Configuration : nesl_utility/Solver Configuration  PhysicalDomain=network_engine_domain  SubClassName=solver  LeftPortType=input  RightPortType=generic  Tones=[]  Harmonics=[]  SimulateNoise=off  Profile=off  UseLocalSampling=off  EnableSwitchedLinearOptims=on  FrequencyDomain=off  UseCCode=off  RelTol=0.001  AbsTol=1e-06  MinStep=1e-09  ToWorkspace=off  RevertToSquareIcSolve=off  NumHomotopyIterations=100  PhasorMode=off  PhasorModeNumHarmonics=1  DoDC=off  ResidualTolerance=1e-9  UseLocalSolver=off  LocalSolverChoice=NE_BACKWARD_EULER_ADVANCER  LocalSolverSampleTime=.001  DoFixedCost=off  MaxNonlinIter=3  MaxModeIter=2  LinearAlgebra=auto  EquationFormulation=NE_TIME_EF  DelaysMemoryBudget=1024  AutomaticFiltering=on  FilteringTimeConstant=0.001  PartitionStorageMethod=AS_NEEDED  PartitionMemoryBudget=1024
  Subsystem : Subsystem
  Out1 : Outport
  wires:
  PS-Simulink/1 -> Out1/1, Display/1
  Subsystem/1(Out1) -> Simulink-PS Converter/1
  In1/1 -> Subsystem/1(In1), Simulink-PS Converter1/1
  connections:
  DC Motor/LConn2 -- Gear Box/LConn1
  Power amplifier/LConn1 -- Controlled Voltage Source/LConn1
  Gear Box/RConn1 -- Ideal Torque Sensor/LConn1
  Controlled Voltage Source1/RConn1 -- Simulink-PS Converter1/RConn1
  DC Motor/RConn2 -- Ideal Torque Sensor/RConn1 -- MRRef/LConn1
  Controlled Voltage Source1/RConn2 -- Power amplifier/LConn3
  DC Motor/RConn1 -- Power amplifier/RConn2 -- Controlled Voltage Source1/LConn1 -- Controlled Voltage Source/RConn2 -- Power amplifier/LConn2 -- Solver Configuration/RConn1 -- ERef/LConn1
  Power amplifier/RConn1 -- DC Motor/LConn1
  Simulink-PS Converter/RConn1 -- Controlled Voltage Source/RConn1
  PS-Simulink/LConn1 -- Ideal Torque Sensor/RConn2

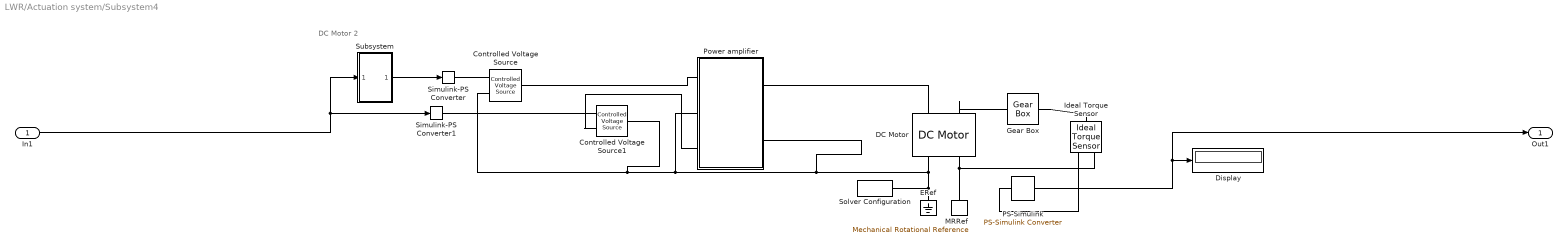
== system LWR/Actuation system/Subsystem4 ==
  note: DC Motor 2
  In1 : Inport
  Controlled Voltage Source : fl_lib/Electrical/Electrical Sources/Controlled Voltage Source
  Controlled Voltage Source1 : fl_lib/Electrical/Electrical Sources/Controlled Voltage Source
  DC Motor : elec_lib/Actuators & Drivers/Rotational Actuators/DC Motor  parameterization=1  Ra=3.38 Ohm  La=0.01 H  emf_or_torque=2  Kv=0.029 V/(rad/s)  Ki=0.638 N*m/A  T_stall=0.1 N*m  w_max=4000 rpm  w_rated=2500 rpm  P_rated=10 W  V_rated=12 V  J=0.2 kg*m^2  lam_param=1  lam=0.5e-5 N*m/(rad/s)  i_noload=0 A  V_i_noload=1.5 V  speed0=0 rpm  alpha=0.00393 1/K  Tmeas=25 degC  thermal_mass=100 J/K  initial_temperature=25 degC
  Display : Display
  ERef : fl_lib/Electrical/Electrical Elements/Electrical Reference
      settings: SourceProductName=Foundation Library
  Gear Box : fl_lib/Mechanical/Mechanisms/Gear Box  ratio=4  t_in_specify=off  t_in_priority=None  t_in=0 N*m  t_in_nominal_specify=off  t_in_nominal_unit=N*m  t_in_nominal_value=1  t_out_specify=off  t_out_priority=None  t_out=0 N*m  t_out_nominal_specify=off  t_out_nominal_unit=N*m  t_out_nominal_value=1
  Ideal Torque Sensor : fl_lib/Mechanical/Mechanical Sensors/Ideal Torque Sensor
  MRRef : fl_lib/Mechanical/Rotational Elements/Mechanical Rotational Reference
      settings: SourceProductName=Foundation Library
  PS-Simulink : nesl_utility/PS-Simulink Converter  PhysicalDomain=network_engine_domain  SubClassName=ps_output  LeftPortType=input  RightPortType=output  PseudoPeriodic=off  Frequencies=[]  Unit=N*m  AffineConversion=off
  Power amplifier : Subsystem
  Simulink-PS Converter : nesl_utility/Simulink-PS Converter  PhysicalDomain=network_engine_domain  SubClassName=ps_input  LeftPortType=input  RightPortType=output  PseudoPeriodic=off  Frequencies=[]  NoiseDistribution=none  NoiseParameters=[]  Unit=V  AffineConversion=off  FilteringAndDerivatives=provide  SimscapeFilterOrder=1  InputFilterTimeConstant=0.001  UdotUserProvided=0
  Simulink-PS Converter1 : nesl_utility/Simulink-PS Converter  PhysicalDomain=network_engine_domain  SubClassName=ps_input  LeftPortType=input  RightPortType=output  PseudoPeriodic=off  Frequencies=[]  NoiseDistribution=none  NoiseParameters=[]  Unit=V  AffineConversion=off  FilteringAndDerivatives=provide  SimscapeFilterOrder=1  InputFilterTimeConstant=0.001  UdotUserProvided=0
  Solver Configuration : nesl_utility/Solver Configuration  PhysicalDomain=network_engine_domain  SubClassName=solver  LeftPortType=input  RightPortType=generic  Tones=[]  Harmonics=[]  SimulateNoise=off  Profile=off  UseLocalSampling=off  EnableSwitchedLinearOptims=on  FrequencyDomain=off  UseCCode=off  RelTol=0.001  AbsTol=1e-06  MinStep=1e-09  ToWorkspace=off  RevertToSquareIcSolve=off  NumHomotopyIterations=100  PhasorMode=off  PhasorModeNumHarmonics=1  DoDC=off  ResidualTolerance=1e-9  UseLocalSolver=off  LocalSolverChoice=NE_BACKWARD_EULER_ADVANCER  LocalSolverSampleTime=.001  DoFixedCost=off  MaxNonlinIter=3  MaxModeIter=2  LinearAlgebra=auto  EquationFormulation=NE_TIME_EF  DelaysMemoryBudget=1024  AutomaticFiltering=on  FilteringTimeConstant=0.001  PartitionStorageMethod=AS_NEEDED  PartitionMemoryBudget=1024
  Subsystem : Subsystem
  Out1 : Outport
  wires:
  PS-Simulink/1 -> Out1/1, Display/1
  Subsystem/1(Out1) -> Simulink-PS Converter/1
  In1/1 -> Subsystem/1(In1), Simulink-PS Converter1/1
  connections:
  DC Motor/LConn2 -- Gear Box/LConn1
  Power amplifier/LConn1 -- Controlled Voltage Source/LConn1
  Gear Box/RConn1 -- Ideal Torque Sensor/LConn1
  Controlled Voltage Source1/RConn1 -- Simulink-PS Converter1/RConn1
  DC Motor/RConn2 -- Ideal Torque Sensor/RConn1 -- MRRef/LConn1
  Controlled Voltage Source1/RConn2 -- Power amplifier/LConn3
  Power amplifier/RConn2 -- Controlled Voltage Source1/LConn1 -- Controlled Voltage Source/RConn2 -- Power amplifier/LConn2 -- DC Motor/RConn1 -- Solver Configuration/RConn1 -- ERef/LConn1
  Simulink-PS Converter/RConn1 -- Controlled Voltage Source/RConn1
  PS-Simulink/LConn1 -- Ideal Torque Sensor/RConn2
  Power amplifier/RConn1 -- DC Motor/LConn1

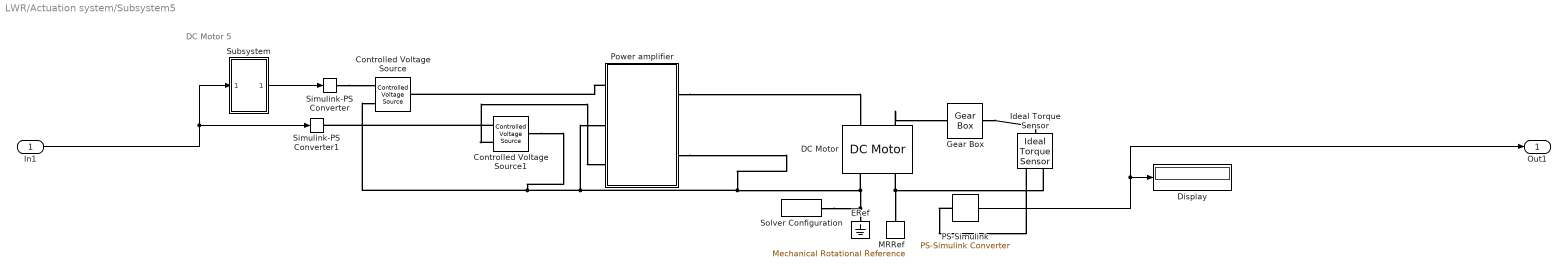
== system LWR/Actuation system/Subsystem5 ==
  note: DC Motor 5
  In1 : Inport
  Controlled Voltage Source : fl_lib/Electrical/Electrical Sources/Controlled Voltage Source
  Controlled Voltage Source1 : fl_lib/Electrical/Electrical Sources/Controlled Voltage Source
  DC Motor : elec_lib/Actuators & Drivers/Rotational Actuators/DC Motor  parameterization=1  Ra=3.38 Ohm  La=0.01 H  emf_or_torque=2  Kv=0.029 V/(rad/s)  Ki=0.638 N*m/A  T_stall=0.1 N*m  w_max=4000 rpm  w_rated=2500 rpm  P_rated=10 W  V_rated=12 V  J=0.2 kg*m^2  lam_param=1  lam=0.5e-5 N*m/(rad/s)  i_noload=0 A  V_i_noload=1.5 V  speed0=0 rpm  alpha=0.00393 1/K  Tmeas=25 degC  thermal_mass=100 J/K  initial_temperature=25 degC
  Display : Display
  ERef : fl_lib/Electrical/Electrical Elements/Electrical Reference
      settings: SourceProductName=Foundation Library
  Gear Box : fl_lib/Mechanical/Mechanisms/Gear Box  ratio=2.5  t_in_specify=off  t_in_priority=None  t_in=0 N*m  t_in_nominal_specify=off  t_in_nominal_unit=N*m  t_in_nominal_value=1  t_out_specify=off  t_out_priority=None  t_out=0 N*m  t_out_nominal_specify=off  t_out_nominal_unit=N*m  t_out_nominal_value=1
  Ideal Torque Sensor : fl_lib/Mechanical/Mechanical Sensors/Ideal Torque Sensor
  MRRef : fl_lib/Mechanical/Rotational Elements/Mechanical Rotational Reference
      settings: SourceProductName=Foundation Library
  PS-Simulink : nesl_utility/PS-Simulink Converter  PhysicalDomain=network_engine_domain  SubClassName=ps_output  LeftPortType=input  RightPortType=output  PseudoPeriodic=off  Frequencies=[]  Unit=N*m  AffineConversion=off
  Power amplifier : Subsystem
  Simulink-PS Converter : nesl_utility/Simulink-PS Converter  PhysicalDomain=network_engine_domain  SubClassName=ps_input  LeftPortType=input  RightPortType=output  PseudoPeriodic=off  Frequencies=[]  NoiseDistribution=none  NoiseParameters=[]  Unit=V  AffineConversion=off  FilteringAndDerivatives=provide  SimscapeFilterOrder=1  InputFilterTimeConstant=0.001  UdotUserProvided=0
  Simulink-PS Converter1 : nesl_utility/Simulink-PS Converter  PhysicalDomain=network_engine_domain  SubClassName=ps_input  LeftPortType=input  RightPortType=output  PseudoPeriodic=off  Frequencies=[]  NoiseDistribution=none  NoiseParameters=[]  Unit=V  AffineConversion=off  FilteringAndDerivatives=provide  SimscapeFilterOrder=1  InputFilterTimeConstant=0.001  UdotUserProvided=0
  Solver Configuration : nesl_utility/Solver Configuration  PhysicalDomain=network_engine_domain  SubClassName=solver  LeftPortType=input  RightPortType=generic  Tones=[]  Harmonics=[]  SimulateNoise=off  Profile=off  UseLocalSampling=off  EnableSwitchedLinearOptims=on  FrequencyDomain=off  UseCCode=off  RelTol=0.001  AbsTol=1e-06  MinStep=1e-09  ToWorkspace=off  RevertToSquareIcSolve=off  NumHomotopyIterations=100  PhasorMode=off  PhasorModeNumHarmonics=1  DoDC=off  ResidualTolerance=1e-9  UseLocalSolver=off  LocalSolverChoice=NE_BACKWARD_EULER_ADVANCER  LocalSolverSampleTime=.001  DoFixedCost=off  MaxNonlinIter=3  MaxModeIter=2  LinearAlgebra=auto  EquationFormulation=NE_TIME_EF  DelaysMemoryBudget=1024  AutomaticFiltering=on  FilteringTimeConstant=0.001  PartitionStorageMethod=AS_NEEDED  PartitionMemoryBudget=1024
  Subsystem : Subsystem
  Out1 : Outport
  wires:
  PS-Simulink/1 -> Out1/1, Display/1
  Subsystem/1(Out1) -> Simulink-PS Converter/1
  In1/1 -> Subsystem/1(In1), Simulink-PS Converter1/1
  connections:
  DC Motor/LConn2 -- Gear Box/LConn1
  Power amplifier/LConn1 -- Controlled Voltage Source/LConn1
  Gear Box/RConn1 -- Ideal Torque Sensor/LConn1
  Controlled Voltage Source1/RConn1 -- Simulink-PS Converter1/RConn1
  DC Motor/RConn2 -- Ideal Torque Sensor/RConn1 -- MRRef/LConn1
  Controlled Voltage Source1/RConn2 -- Power amplifier/LConn3
  DC Motor/RConn1 -- Power amplifier/RConn2 -- Controlled Voltage Source1/LConn1 -- Controlled Voltage Source/RConn2 -- Power amplifier/LConn2 -- Solver Configuration/RConn1 -- ERef/LConn1
  Power amplifier/RConn1 -- DC Motor/LConn1
  Simulink-PS Converter/RConn1 -- Controlled Voltage Source/RConn1
  PS-Simulink/LConn1 -- Ideal Torque Sensor/RConn2

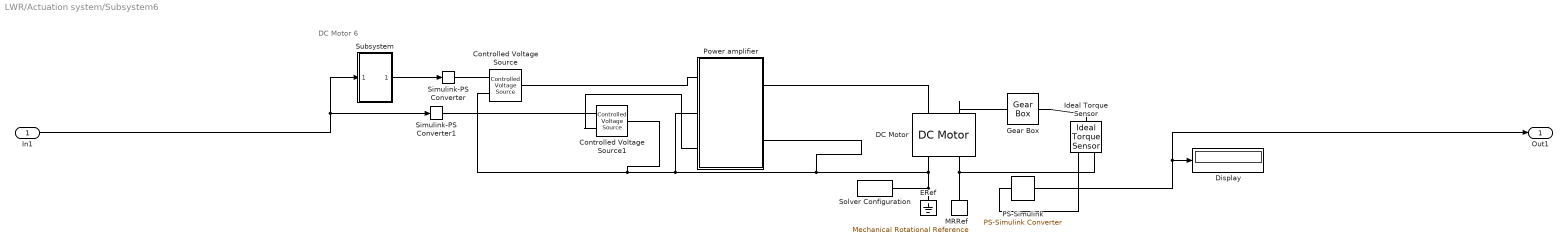
== system LWR/Actuation system/Subsystem6 ==
  note: DC Motor 6
  In1 : Inport
  Controlled Voltage Source : fl_lib/Electrical/Electrical Sources/Controlled Voltage Source
  Controlled Voltage Source1 : fl_lib/Electrical/Electrical Sources/Controlled Voltage Source
  DC Motor : elec_lib/Actuators & Drivers/Rotational Actuators/DC Motor  parameterization=1  Ra=3.38 Ohm  La=0.01 H  emf_or_torque=2  Kv=0.029 V/(rad/s)  Ki=0.638 N*m/A  T_stall=0.1 N*m  w_max=4000 rpm  w_rated=2500 rpm  P_rated=10 W  V_rated=12 V  J=0.2 kg*m^2  lam_param=1  lam=0.5e-5 N*m/(rad/s)  i_noload=0 A  V_i_noload=1.5 V  speed0=0 rpm  alpha=0.00393 1/K  Tmeas=25 degC  thermal_mass=100 J/K  initial_temperature=25 degC
  Display : Display
  ERef : fl_lib/Electrical/Electrical Elements/Electrical Reference
      settings: SourceProductName=Foundation Library
  Gear Box : fl_lib/Mechanical/Mechanisms/Gear Box  ratio=0.9  t_in_specify=off  t_in_priority=None  t_in=0 N*m  t_in_nominal_specify=off  t_in_nominal_unit=N*m  t_in_nominal_value=1  t_out_specify=off  t_out_priority=None  t_out=0 N*m  t_out_nominal_specify=off  t_out_nominal_unit=N*m  t_out_nominal_value=1
  Ideal Torque Sensor : fl_lib/Mechanical/Mechanical Sensors/Ideal Torque Sensor
  MRRef : fl_lib/Mechanical/Rotational Elements/Mechanical Rotational Reference
      settings: SourceProductName=Foundation Library
  PS-Simulink : nesl_utility/PS-Simulink Converter  PhysicalDomain=network_engine_domain  SubClassName=ps_output  LeftPortType=input  RightPortType=output  PseudoPeriodic=off  Frequencies=[]  Unit=N*m  AffineConversion=off
  Power amplifier : Subsystem
  Simulink-PS Converter : nesl_utility/Simulink-PS Converter  PhysicalDomain=network_engine_domain  SubClassName=ps_input  LeftPortType=input  RightPortType=output  PseudoPeriodic=off  Frequencies=[]  NoiseDistribution=none  NoiseParameters=[]  Unit=V  AffineConversion=off  FilteringAndDerivatives=provide  SimscapeFilterOrder=1  InputFilterTimeConstant=0.001  UdotUserProvided=0
  Simulink-PS Converter1 : nesl_utility/Simulink-PS Converter  PhysicalDomain=network_engine_domain  SubClassName=ps_input  LeftPortType=input  RightPortType=output  PseudoPeriodic=off  Frequencies=[]  NoiseDistribution=none  NoiseParameters=[]  Unit=V  AffineConversion=off  FilteringAndDerivatives=provide  SimscapeFilterOrder=1  InputFilterTimeConstant=0.001  UdotUserProvided=0
  Solver Configuration : nesl_utility/Solver Configuration  PhysicalDomain=network_engine_domain  SubClassName=solver  LeftPortType=input  RightPortType=generic  Tones=[]  Harmonics=[]  SimulateNoise=off  Profile=off  UseLocalSampling=off  EnableSwitchedLinearOptims=on  FrequencyDomain=off  UseCCode=off  RelTol=0.001  AbsTol=1e-06  MinStep=1e-09  ToWorkspace=off  RevertToSquareIcSolve=off  NumHomotopyIterations=100  PhasorMode=off  PhasorModeNumHarmonics=1  DoDC=off  ResidualTolerance=1e-9  UseLocalSolver=off  LocalSolverChoice=NE_BACKWARD_EULER_ADVANCER  LocalSolverSampleTime=.001  DoFixedCost=off  MaxNonlinIter=3  MaxModeIter=2  LinearAlgebra=auto  EquationFormulation=NE_TIME_EF  DelaysMemoryBudget=1024  AutomaticFiltering=on  FilteringTimeConstant=0.001  PartitionStorageMethod=AS_NEEDED  PartitionMemoryBudget=1024
  Subsystem : Subsystem
  Out1 : Outport
  wires:
  PS-Simulink/1 -> Out1/1, Display/1
  Subsystem/1(Out1) -> Simulink-PS Converter/1
  In1/1 -> Subsystem/1(In1), Simulink-PS Converter1/1
  connections:
  DC Motor/LConn2 -- Gear Box/LConn1
  Power amplifier/LConn1 -- Controlled Voltage Source/LConn1
  Gear Box/RConn1 -- Ideal Torque Sensor/LConn1
  Controlled Voltage Source1/RConn1 -- Simulink-PS Converter1/RConn1
  DC Motor/RConn2 -- Ideal Torque Sensor/RConn1 -- MRRef/LConn1
  Controlled Voltage Source1/RConn2 -- Power amplifier/LConn3
  DC Motor/RConn1 -- Power amplifier/RConn2 -- Controlled Voltage Source1/LConn1 -- Controlled Voltage Source/RConn2 -- Power amplifier/LConn2 -- Solver Configuration/RConn1 -- ERef/LConn1
  Power amplifier/RConn1 -- DC Motor/LConn1
  Simulink-PS Converter/RConn1 -- Controlled Voltage Source/RConn1
  PS-Simulink/LConn1 -- Ideal Torque Sensor/RConn2

== system LWR/Actuation system/Subsystem7 ==
  note: DC Motor 7
  In1 : Inport
  Controlled Voltage Source : fl_lib/Electrical/Electrical Sources/Controlled Voltage Source
  Controlled Voltage Source1 : fl_lib/Electrical/Electrical Sources/Controlled Voltage Source
  DC Motor : elec_lib/Actuators & Drivers/Rotational Actuators/DC Motor  parameterization=1  Ra=3.38 Ohm  La=0.01 H  emf_or_torque=2  Kv=0.029 V/(rad/s)  Ki=0.638 N*m/A  T_stall=0.1 N*m  w_max=4000 rpm  w_rated=2500 rpm  P_rated=10 W  V_rated=12 V  J=0.2 kg*m^2  lam_param=1  lam=0.5e-5 N*m/(rad/s)  i_noload=0 A  V_i_noload=1.5 V  speed0=0 rpm  alpha=0.00393 1/K  Tmeas=25 degC  thermal_mass=100 J/K  initial_temperature=25 degC
  Display : Display
  ERef : fl_lib/Electrical/Electrical Elements/Electrical Reference
      settings: SourceProductName=Foundation Library
  Gear Box : fl_lib/Mechanical/Mechanisms/Gear Box  ratio=0.9  t_in_specify=off  t_in_priority=None  t_in=0 N*m  t_in_nominal_specify=off  t_in_nominal_unit=N*m  t_in_nominal_value=1  t_out_specify=off  t_out_priority=None  t_out=0 N*m  t_out_nominal_specify=off  t_out_nominal_unit=N*m  t_out_nominal_value=1
  Ideal Torque Sensor : fl_lib/Mechanical/Mechanical Sensors/Ideal Torque Sensor
  MRRef : fl_lib/Mechanical/Rotational Elements/Mechanical Rotational Reference
      settings: SourceProductName=Foundation Library
  PS-Simulink : nesl_utility/PS-Simulink Converter  PhysicalDomain=network_engine_domain  SubClassName=ps_output  LeftPortType=input  RightPortType=output  PseudoPeriodic=off  Frequencies=[]  Unit=N*m  AffineConversion=off
  Power amplifier : Subsystem
  Simulink-PS Converter : nesl_utility/Simulink-PS Converter  PhysicalDomain=network_engine_domain  SubClassName=ps_input  LeftPortType=input  RightPortType=output  PseudoPeriodic=off  Frequencies=[]  NoiseDistribution=none  NoiseParameters=[]  Unit=V  AffineConversion=off  FilteringAndDerivatives=provide  SimscapeFilterOrder=1  InputFilterTimeConstant=0.001  UdotUserProvided=0
  Simulink-PS Converter1 : nesl_utility/Simulink-PS Converter  PhysicalDomain=network_engine_domain  SubClassName=ps_input  LeftPortType=input  RightPortType=output  PseudoPeriodic=off  Frequencies=[]  NoiseDistribution=none  NoiseParameters=[]  Unit=V  AffineConversion=off  FilteringAndDerivatives=provide  SimscapeFilterOrder=1  InputFilterTimeConstant=0.001  UdotUserProvided=0
  Solver Configuration : nesl_utility/Solver Configuration  PhysicalDomain=network_engine_domain  SubClassName=solver  LeftPortType=input  RightPortType=generic  Tones=[]  Harmonics=[]  SimulateNoise=off  Profile=off  UseLocalSampling=off  EnableSwitchedLinearOptims=on  FrequencyDomain=off  UseCCode=off  RelTol=0.001  AbsTol=1e-06  MinStep=1e-09  ToWorkspace=off  RevertToSquareIcSolve=off  NumHomotopyIterations=100  PhasorMode=off  PhasorModeNumHarmonics=1  DoDC=off  ResidualTolerance=1e-9  UseLocalSolver=off  LocalSolverChoice=NE_BACKWARD_EULER_ADVANCER  LocalSolverSampleTime=.001  DoFixedCost=off  MaxNonlinIter=3  MaxModeIter=2  LinearAlgebra=auto  EquationFormulation=NE_TIME_EF  DelaysMemoryBudget=1024  AutomaticFiltering=on  FilteringTimeConstant=0.001  PartitionStorageMethod=AS_NEEDED  PartitionMemoryBudget=1024
  Subsystem : Subsystem
  Out1 : Outport
  wires:
  PS-Simulink/1 -> Out1/1, Display/1
  Subsystem/1(Out1) -> Simulink-PS Converter/1
  In1/1 -> Subsystem/1(In1), Simulink-PS Converter1/1
  connections:
  DC Motor/LConn2 -- Gear Box/LConn1
  Power amplifier/LConn1 -- Controlled Voltage Source/LConn1
  Gear Box/RConn1 -- Ideal Torque Sensor/LConn1
  Controlled Voltage Source1/RConn1 -- Simulink-PS Converter1/RConn1
  DC Motor/RConn2 -- Ideal Torque Sensor/RConn1 -- MRRef/LConn1
  Controlled Voltage Source1/RConn2 -- Power amplifier/LConn3
  DC Motor/RConn1 -- Power amplifier/RConn2 -- Controlled Voltage Source1/LConn1 -- Controlled Voltage Source/RConn2 -- Power amplifier/LConn2 -- Solver Configuration/RConn1 -- ERef/LConn1
  Power amplifier/RConn1 -- DC Motor/LConn1
  Simulink-PS Converter/RConn1 -- Controlled Voltage Source/RConn1
  PS-Simulink/LConn1 -- Ideal Torque Sensor/RConn2

== system LWR/Controller/SMC 1 ==
  note: Maximum output
  note: Sliding surface
  note: Gain
  error : Inport
  Alpha : Constant  Value=7.5
  Derivative : Derivative  CoefficientInTFapproximation=0.01
  Gamma : Constant  Value=0.04
  Lambda : Constant  Value=5
  Multiply : Product
  Multiply1 : Product
  Multiply2 : Product
  Sum1 : Sum
  Tanh : Trigonometry  Operator=tanh
  Out1 : Outport
  wires:
  Gamma/1 -> Multiply2/1
  Multiply/1 -> Sum1/1
  Tanh/1 -> Multiply1/1
  Lambda/1 -> Multiply1/2
  Alpha/1 -> Multiply/1
  Sum1/1 -> Multiply2/2
  error/1 -> Multiply/2, Derivative/1
  Multiply2/1 -> Tanh/1
  Derivative/1 -> Sum1/2
  Multiply1/1 -> Out1/1

== system LWR/Controller/SMC 2 ==
  error : Inport
  Alpha : Constant  Value=15
  Derivative : Derivative  CoefficientInTFapproximation=0.01
  Gamma : Constant  Value=0.5
  Lambda : Constant  Value=5
  Multiply : Product
  Multiply1 : Product
  Multiply2 : Product
  Sum1 : Sum
  Tanh : Trigonometry  Operator=tanh
  Out1 : Outport
  wires:
  Gamma/1 -> Multiply2/1
  Multiply/1 -> Sum1/1
  Tanh/1 -> Multiply1/1
  Lambda/1 -> Multiply1/2
  Alpha/1 -> Multiply/1
  Sum1/1 -> Multiply2/2
  error/1 -> Multiply/2, Derivative/1
  Multiply2/1 -> Tanh/1
  Derivative/1 -> Sum1/2
  Multiply1/1 -> Out1/1
